simulink model "mhe_testing"  (R2023b)
settings: Solver=VariableStepAuto  StartTime=0.0  StopTime=30  RelTol=1e-3
settings Model: Creator=akeebismail  LastModifiedBy=akeebismail

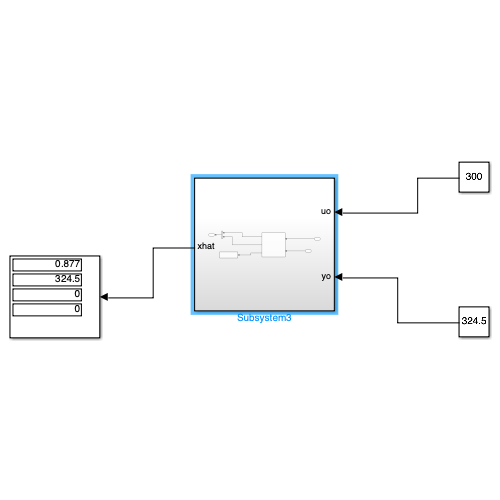
[thumbnail: Simulink's stored preview of the top-level diagram]
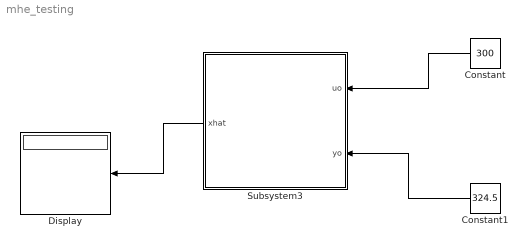
== system mhe_testing ==
  Constant : Constant  Value=300
  Constant1 : Constant  Value=324.5
  Display : Display
  Subsystem3 : Subsystem
  wires:
  Subsystem3/1(xhat) -> Display/1
  Constant/1 -> Subsystem3/1(uo)
  Constant1/1 -> Subsystem3/2(yo)

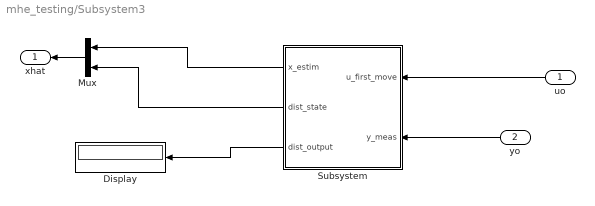
== system mhe_testing/Subsystem3 ==
  uo : Inport
  yo : Inport  Port=2
  Display : Display
  Mux : Mux  Inputs=2
  Subsystem : Subsystem
  xhat : Outport
  wires:
  Subsystem/1(x_estim) -> Mux/1
  Subsystem/2(dist_state) -> Mux/2
  Subsystem/3(dist_output) -> Display/1
  uo/1 -> Subsystem/1(u_first_move)
  yo/1 -> Subsystem/2(y_meas)
  Mux/1 -> xhat/1

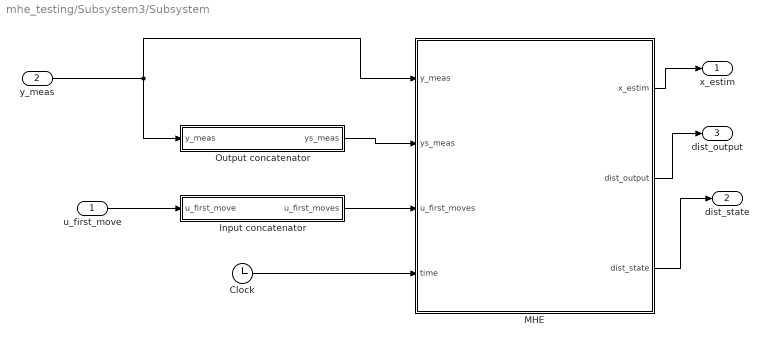
== system mhe_testing/Subsystem3/Subsystem ==
  u_first_move : Inport  PortDimensions=[1,1]
  y_meas : Inport  Port=2  PortDimensions=[1,1]
  Clock : Clock
      settings: Decimation=20
  Input concatenator : Subsystem
  MHE : MATLAB Function  TreatAsAtomicUnit=on
  Output concatenator : Subsystem
  x_estim : Outport
  dist_state : Outport  Port=2
  dist_output : Outport  Port=3
  wires:
  Input concatenator/1(u_first_moves) -> MHE/3(u_first_moves)
  MHE/3(dist_state) -> dist_state/1
  MHE/2(dist_output) -> dist_output/1
  Clock/1 -> MHE/4(time)
  u_first_move/1 -> Input concatenator/1(u_first_move)
  MHE/1(x_estim) -> x_estim/1
  y_meas/1 -> MHE/1(y_meas), Output concatenator/1(y_meas)
  Output concatenator/1(ys_meas) -> MHE/2(ys_meas)

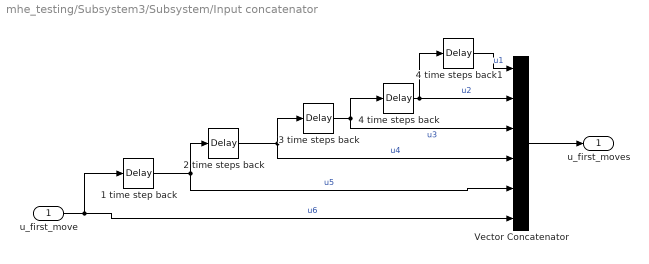
== system mhe_testing/Subsystem3/Subsystem/Input concatenator ==
  u_first_move : Inport
  1 time step back : TransportDelay  DelayTime=0.05  InitialOutput=300
  2 time steps back : TransportDelay  DelayTime=0.05  InitialOutput=300
  3 time steps back : TransportDelay  DelayTime=0.05  InitialOutput=300
  4 time steps back : TransportDelay  DelayTime=0.05  InitialOutput=300
  4 time steps back1 : TransportDelay  DelayTime=0.05  InitialOutput=300
  Vector Concatenator : Concatenate  NumInputs=6  Mode=Multidimensional array
  u_first_moves : Outport  PortDimensions=[6,1]  VectorParamsAs1DForOutWhenUnconnected=off
  wires:
  Vector Concatenator/1 -> u_first_moves/1
  u_first_move/1 -> Vector Concatenator/6, 1 time step back/1  "u6"
  4 time steps back/1 -> Vector Concatenator/2, 4 time steps back1/1  "u2"
  3 time steps back/1 -> Vector Concatenator/3, 4 time steps back/1  "u3"
  2 time steps back/1 -> 3 time steps back/1, Vector Concatenator/4  "u4"
  1 time step back/1 -> 2 time steps back/1, Vector Concatenator/5  "u5"
  4 time steps back1/1 -> Vector Concatenator/1  "u1"

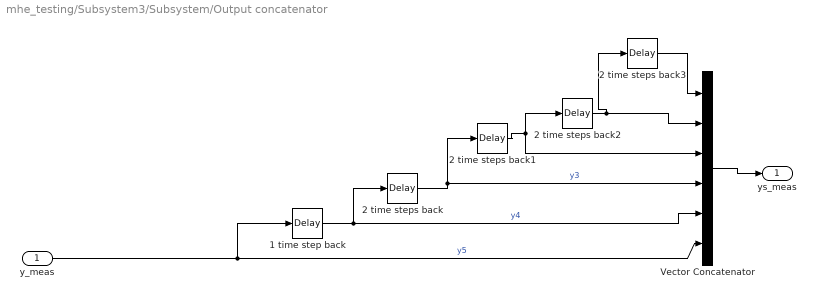
== system mhe_testing/Subsystem3/Subsystem/Output concatenator ==
  y_meas : Inport
  1 time step back : TransportDelay  DelayTime=0.05  InitialOutput=324.5
  2 time steps back{,1..3} (4 alike) : TransportDelay  DelayTime=0.05  InitialOutput=324.5
  Vector Concatenator : Concatenate  NumInputs=6  Mode=Multidimensional array
  ys_meas : Outport  PortDimensions=[6,1]  VectorParamsAs1DForOutWhenUnconnected=off
  wires:
  2 time steps back2/1 -> 2 time steps back3/1, Vector Concatenator/2
  2 time steps back1/1 -> 2 time steps back2/1, Vector Concatenator/3
  Vector Concatenator/1 -> ys_meas/1
  2 time steps back/1 -> 2 time steps back1/1, Vector Concatenator/4  "y3"
  1 time step back/1 -> Vector Concatenator/5, 2 time steps back/1  "y4"
  y_meas/1 -> Vector Concatenator/6, 1 time step back/1  "y5"
  2 time steps back3/1 -> Vector Concatenator/1

== matlab function mhe_testing/Subsystem3/Subsystem/MHE ==
  data: y_meas input; ys_meas input; x_estim output; u_first_moves input; time input; dist_output output; dist_state output
function [x_estim,dist_output,dist_state] = MHE_4_tanks(y_meas,ys_meas,u_first_moves,time)

coder.extrinsic('MHE_compute');

N_MHE=6  ;
% Ts=2 ;


if time < 0.5
    
    x_estim =  [0.877;324.5]  ;
   % x_estim = [17;17;17];
    %x_estim = [5.898;1.8];
    dist_output = 0;
    dist_state = [0;0];
else
    
    [x_estim,dist_state,dist_output] = MHE_compute(ys_meas,u_first_moves,N_MHE,y_meas);
    %Note that our horizon must be constant here. It is chosen as 5.
end

end
